simulink library "ammclib_bam_S32K3xx"  (R2016a)
(part 34 of 50)

      |   SampleTime=Simulink.data.evalinGlobal(bdroot,get_param(gcb,'SampleTime'));
      |   if (SampleTime==-1)
      |     SampleTime=str2double(get_param(gcb,'SampleTime_1'));
      |   end
      |   f16C1_bkup=get_param(gcb,'f16C1');
      |   u16NShift_bkup=get_param(gcb,'u16NShift');
      |   inscale=Simulink.data.evalinGlobal(bdroot,get_param(gcb,'inscale'));
      |   outscale=Simulink.data.evalinGlobal(bdroot,get_param(gcb,'outscale'));
      |   if (inscale<=0)
      |     warning('E_max must be positive.');
      |   end
      |   if (outscale<=0)
      |     warning('U_max must be positive.');
      |   end
      |   c1f=SampleTime*0.5*inscale/outscale;
      |   u16NShift=ceil(log2(abs(c1f)));
      |   if u16NShift<0
      |     u16NShift=0;
      |   end
      |   if u16NShift>15
      |     u16NShift=15;
      |     warning(['Parameter u16NShift of ' gcb ' exceeds the fixed-point range.']);
      |   end
      |   f16C1=round(c1f*2^(-u16NShift)*2^15);
      |   if f16C1>2^15-1
      |     f16C1=2^15-1;
      |     warning(['Parameter f16C1 of ' gcb ' exceeds the fixed-point range.']);
      |   end
      |   if f16C1<-2^15
      |     f16C1=-2^15;
      |     warning(['Parameter f16C1 of ' gcb ' exceeds the fixed-point range.']);
      |   end
      |   if isnan(f16C1)
      |     if ~strcmp(f16C1_bkup,'0')
      |       set_param(gcb,'f16C1','0');
      |     end
      |   else
      |     tmps=num2str(f16C1);
      |     if ~strcmp(f16C1_bkup,tmps)
      |       set_param(gcb,'f16C1',tmps);
      |     end
      |   end
      |   if isnan(u16NShift)
      |     if ~strcmp(u16NShift_bkup,'0')
      |       set_param(gcb,'u16NShift','0');
      |     end
      |   else
      |     tmps=num2str(u16NShift);
      |     if ~strcmp(u16NShift_bkup,tmps)
      |       set_param(gcb,'u16NShift',tmps);
      |     end
      |   end
      | end
      mask Callback autoCalcEn:
      | maskStr=get_param(gcb,'showStates');
      | if strcmp(maskStr,'Hide (faster execution)')
      |   p=Simulink.Mask.get(gcb);
      |   autoCalcEn=get_param(gcb,'autoCalcEn');
      |   hintText=p.getDialogControl('timeHint');
      |   if strcmp(autoCalcEn,'on')
      |     param=p.getParameter('outscale');
      |     if strcmp(param.Enabled,'off')
      |       SampleTime=Simulink.data.evalinGlobal(bdroot,get_param(gcb,'SampleTime'));
      |       if SampleTime==-1
      |         SampleTime=str2double(get_param(gcb,'SampleTime_1'));
      |         if isnan(SampleTime)
      |           hintText.Prompt=['Note: Implementation parameters cannot be calculated yet because the block''s inherited sample time is unknown. Simulink will update the sample time when you run the simulation.'];
      |         else
      |           hintText.Prompt=['Caution: Implementation parameters depend on inherited sample time. Make sure that the sample time of the block''s inputs corresponds to the sampling period in the target application.'];
      |         end
      |       else
      |         hintText.Prompt='Caution: Implementation parameters depend on the sample time. Make sure that the simulation time step corresponds to the sampling period in the target application.';
      |       end
      |       p=Simulink.Mask.get(gcb);
      |       param=p.getParameter('inscale');
      |       param.set('Enabled','on');
      |       param=p.getParameter('outscale');
      |       param.set('Enabled','on');
      |     else
      |       SampleTime=Simulink.data.evalinGlobal(bdroot,get_param(gcb,'SampleTime'));
      |       if SampleTime==-1
      |         SampleTime=str2double(get_param(gcb,'SampleTime_1'));
      |       end
      |     end
      |     f16C1_bkup=get_param(gcb,'f16C1');
      |     u16NShift_bkup=get_param(gcb,'u16NShift');
      |     inscale=Simulink.data.evalinGlobal(bdroot,get_param(gcb,'inscale'));
      |     outscale=Simulink.data.evalinGlobal(bdroot,get_param(gcb,'outscale'));
      |     if (inscale<=0)
      |       warning('E_max must be positive.');
      |     end
      |     if (outscale<=0)
      |       warning('U_max must be positive.');
      |     end
      |     c1f=SampleTime*0.5*inscale/outscale;
      |     u16NShift=ceil(log2(abs(c1f)));
      |     if u16NShift<0
      |       u16NShift=0;
      |     end
      |     if u16NShift>15
      |       u16NShift=15;
      |       warning(['Parameter u16NShift of ' gcb ' exceeds the fixed-point range.']);
      |     end
      |     f16C1=round(c1f*2^(-u16NShift)*2^15);
      |     if f16C1>2^15-1
      |       f16C1=2^15-1;
      |       warning(['Parameter f16C1 of ' gcb ' exceeds the fixed-point range.']);
      |     end
      |     if f16C1<-2^15
      |       f16C1=-2^15;
      |       warning(['Parameter f16C1 of ' gcb ' exceeds the fixed-point range.']);
      |     end
      |     if isnan(f16C1)
      |       if ~strcmp(f16C1_bkup,'0')
      |         set_param(gcb,'f16C1','0');
      |       end
      |     else
      |       tmps=num2str(f16C1);
      |       if ~strcmp(f16C1_bkup,tmps)
      |         set_param(gcb,'f16C1',tmps);
      |       end
      |     end
      |     if isnan(u16NShift)
      |       if ~strcmp(u16NShift_bkup,'0')
      |         set_param(gcb,'u16NShift','0');
      |       end
      |     else
      |       tmps=num2str(u16NShift);
      |       if ~strcmp(u16NShift_bkup,tmps)
      |         set_param(gcb,'u16NShift',tmps);
      |       end
      |     end
      |   else
      |     param=p.getParameter('outscale');
      |     if strcmp(param.Enabled,'on')
      |       hintText.Prompt='Caution: Implementation parameters are fixed.';
      |       p=Simulink.Mask.get(gcb);
      |       param=p.getParameter('inscale');
      |       param.set('Enabled','off');
      |       param=p.getParameter('outscale');
      |       param.set('Enabled','off');
      |     end
      |   end
      | end
      mask DialogControl CompBut Prompt: Recalculate sample times
      mask DialogControl CompBut Tooltip: Simulink updates the sample times of all blocks when the simulation is run. This button will update the sample times now.
      mask DialogControl CompBut Callback:
      | btn=questdlg('This will apply all changes in all open dialog boxes and update the schematic. Do you want to proceed?','Apply all changes','Continue','Cancel','Continue');
      | if strcmp(btn,'Continue')
      |   dlgs=DAStudio.ToolRoot.getOpenDialogs;
      |   for i=1:length(dlgs)
      |     dlgs(i).apply;
      |   end
      |   try
      |     SampleTime_1=str2double(get_param(gcb,'SampleTime_1'));
      |     ts=Simulink.Block.getSampleTimes(gcb);
      |     ts=ts(1).Value(1);
      |     if (SampleTime_1 ~= ts)
      |       SampleTime_1=ts;
      |       set_param(gcb,'SampleTime_1',num2str(ts));
      |       autoCalcEn=get_param(gcb,'autoCalcEn');
      |       if strcmp(autoCalcEn,'on')
      |         SampleTime=Simulink.data.evalinGlobal(bdroot,get_param(gcb,'SampleTime'));
      |         p=Simulink.Mask.get(gcb);
      |         hintText=p.getDialogControl('timeHint');
      |         if SampleTime==-1
      |           SampleTime=SampleTime_1;
      |           hintText.Prompt='Caution: Implementation parameters depend on inherited sample time. Make sure that the sample time of the block''s inputs corresponds to the sampling period in the target application.';
      |         else
      |           hintText.Prompt='Caution: Implementation parameters depend on the sample time. Make sure that the simulation time step corresponds to the sampling period in the target application.';
      |         end
      |         f16C1_bkup=get_param(gcb,'f16C1');
      |         u16NShift_bkup=get_param(gcb,'u16NShift');
      |         inscale=Simulink.data.evalinGlobal(bdroot,get_param(gcb,'inscale'));
      |         outscale=Simulink.data.evalinGlobal(bdroot,get_param(gcb,'outscale'));
      |         if (inscale<=0)
      |           warning('E_max must be positive.');
      |         end
      |         if (outscale<=0)
      |           warning('U_max must be positive.');
      |         end
      |         c1f=SampleTime*0.5*inscale/outscale;
      |         u16NShift=ceil(log2(abs(c1f)));
      |         if u16NShift<0
      |           u16NShift=0;
      |         end
      |         if u16NShift>15
      |           u16NShift=15;
      |           warning(['Parameter u16NShift of ' gcb ' exceeds the fixed-point range.']);
      |         end
      |         f16C1=round(c1f*2^(-u16NShift)*2^15);
      |         if f16C1>2^15-1
      |           f16C1=2^15-1;
      |           warning(['Parameter f16C1 of ' gcb ' exceeds the fixed-point range.']);
      |         end
      |         if f16C1<-2^15
      |           f16C1=-2^15;
      |           warning(['Parameter f16C1 of ' gcb ' exceeds the fixed-point range.']);
      |         end
      |         if isnan(f16C1)
      |           if ~strcmp(f16C1_bkup,'0')
      |             set_param(gcb,'f16C1','0');
      |           end
      |         else
      |           tmps=num2str(f16C1);
      |           if ~strcmp(f16C1_bkup,tmps)
      |             set_param(gcb,'f16C1',tmps);
      |           end
      |         end
      |         if isnan(u16NShift)
      |           if ~strcmp(u16NShift_bkup,'0')
      |             set_param(gcb,'u16NShift','0');
      |           end
      |         else
      |           tmps=num2str(u16NShift);
      |           if ~strcmp(u16NShift_bkup,tmps)
      |             set_param(gcb,'u16NShift',tmps);
      |           end
      |         end
      |       end
      |     end
      |   catch
      |    warning(['Sample time cannot be calculated for the block ' gcb])
      |   end
      | end
      mask DialogControl timeHint Prompt: Note: Implementation parameters cannot be calculated yet because the block's inherited sample time is unknown. Simulink will update the sample time when you run the simulation.
      mask Display:
      | color('black');
      | pos = get_param(gcb, 'Position');
      | width = pos(3) - pos(1);
      | height = pos(4) - pos(2);
      | tX=width/2;
      | tY=height - 25;
      | color('black');
      | text(tX,tY, 'GFLIB_IntegratorTR_F16', 'horizontalAlignment', 'center');
      | if showStates == 2
      |   color('red');
      |   text(tX,tY - 20, ['debugging mode' char(13) char(10) '(limited performance)'], 'horizontalAlignment', 'center');
      | end
  GFLIB_Limit_F16 : Subsystem  TreatAsAtomicUnit=on  mask(GFLIB_Limit_F16){showStates=Hide (faster execution), f16LowerLimit=0, f16UpperLimit=0}
      mask prompts: showStates "Show parameters as inputs:"; f16LowerLimit "f16LowerLimit (Lower limit):"; f16UpperLimit "f16UpperLimit (Upper limit):"
      mask help: Limit function in 16-bit fixed-point fractional implementation. Refer to the AMMCLIB User's Guide for further details.
      mask init:
      | ddName = get_param(bdroot,'DataDictionary');
      | if length(ddName)==0
      |   set_param(bdroot,'DataDictionary','ammclib_types.sldd');
      | else
      |   dd = Simulink.data.dictionary.open(ddName);
      |   data = getSection(dd,'Design Data');
      |   if ~exist(data,'SWLIBS_2Syst_F16')
      |     addDataSource(dd,'ammclib_types.sldd');
      |     saveChanges(dd);
      |   end
      | end
      | 
      | if showStates == 1
      |   % hidden state variables
      |   if strcmp(get_param([gcb '/f16LowerLimit'], 'BlockType'), 'Inport')
      |     posblk = get_param(gcb, 'Position');
      | 
      |     pos = get_param([gcb, '/f16LowerLimit'], 'Position');
      |     orient = get_param([gcb, '/f16LowerLimit'], 'Orientation');
      |     delete_block([gcb, '/f16LowerLimit']);
      |     add_block('built-in/Ground', [gcb, '/f16LowerLimit'], 'Position', pos, 'Orientation', orient);
      | 
      |     pos = get_param([gcb, '/f16UpperLimit'], 'Position');
      |     orient = get_param([gcb, '/f16UpperLimit'], 'Orientation');
      |     delete_block([gcb, '/f16UpperLimit']);
      |     add_block('built-in/Ground', [gcb, '/f16UpperLimit'], 'Position', pos, 'Orientation', orient);
      | 
      | 
      |     set_param([gcb '/f16In'], 'Port', '1');
      | 
      |     tmpOutCnt=0;
      |     tmpOutCnt=tmpOutCnt+1;
      |     set_param([gcb '/f16Out'], 'Port', num2str(tmpOutCnt));
      | 
      | set_param(gcb,'MaskEnables',{'on','on','on'});
      | 
      |     if (posblk(4) - posblk(2)) > 50
      |       height = 50;
      |       set_param(gcb,'Position',[posblk(1), posblk(2), posblk(3), posblk(2)+height])
      |     end
      |   end
      | else
      |   % shown state variables
      |   if strcmp(get_param([gcb '/f16LowerLimit'], 'BlockType'), 'Ground')
      |     posblk = get_param(gcb, 'Position');
      | 
      |     pos = get_param([gcb, '/f16LowerLimit'], 'Position');
      |     orient = get_param([gcb, '/f16LowerLimit'], 'Orientation');
      |     delete_block([gcb, '/f16LowerLimit']);
      |     add_block('built-in/Inport', [gcb, '/f16LowerLimit'], 'Position', pos, 'Orientation', orient, 'OutDataTypeStr', 'int16');
      | 
      |     pos = get_param([gcb, '/f16UpperLimit'], 'Position');
      |     orient = get_param([gcb, '/f16UpperLimit'], 'Orientation');
      |     delete_block([gcb, '/f16UpperLimit']);
      |     add_block('built-in/Inport', [gcb, '/f16UpperLimit'], 'Position', pos, 'Orientation', orient, 'OutDataTypeStr', 'int16');
      | 
      | 
      | 
      | 
      |     set_param([gcb '/f16In'], 'Port', '1');
      |     set_param([gcb '/f16LowerLimit'], 'Port', '2');
      |     set_param([gcb '/f16UpperLimit'], 'Port', '3');
      | 
      |     tmpOutCnt=0;
      |     tmpOutCnt=tmpOutCnt+1;
      |     set_param([gcb '/f16Out'], 'Port', num2str(tmpOutCnt));
      | 
      |     set_param(gcb,'MaskEnables',{'on','off','off'});
      | 
      |     if (posblk(4) - posblk(2)) < 100
      |       height = 100;
      |       set_param(gcb,'Position',[posblk(1), posblk(2), posblk(3), posblk(2)+height])
      |     end
      |   end
      | end
      settings: RTWSystemCode=Inline
      mask Help: web([fileparts(which('ammclib_bam_S32K3xx.slx')) '/../doc/S32K3XXMCLUG.pdf'], '-browser')
      mask TypeOptions showStates: Hide (faster execution) | Show (parameters can be changed during simulation)
      mask Callback showStates:
      | maskStr=get_param(gcb,'showStates');
      | if strcmp(maskStr,'Hide (faster execution)')
      |   if strcmp(get_param([gcb '/f16LowerLimit'], 'BlockType'), 'Inport')
      | set_param(gcb,'MaskEnables',{'on','on','on'});
      |   end
      | else
      |   if strcmp(get_param([gcb '/f16LowerLimit'], 'BlockType'), 'Ground')
      |     set_param(gcb,'MaskEnables',{'on','off','off'});
      |   end
      | end
      mask Display:
      | color('black');
      | pos = get_param(gcb, 'Position');
      | width = pos(3) - pos(1);
      | height = pos(4) - pos(2);
      | tX=width/2;
      | tY=height - 8;
      | color('black');
      | text(tX,tY, 'GFLIB_Limit_F16', 'horizontalAlignment', 'center');
      | if showStates == 2
      |   color('red');
      |   text(tX,tY - 20, ['debugging mode' char(13) char(10) '(limited performance)'], 'horizontalAlignment', 'center');
      | end
  GFLIB_LowerLimit_F16 : Subsystem  TreatAsAtomicUnit=on  mask(GFLIB_LowerLimit_F16){showStates=Hide (faster execution), f16LowerLimit=0}
      mask prompts: showStates "Show parameters as inputs:"; f16LowerLimit "f16LowerLimit (Value determining the lower limit threshold):"
      mask help: Lower limit function in 16-bit fixed-point fractional implementation. Refer to the AMMCLIB User's Guide for further details.
      mask init:
      | ddName = get_param(bdroot,'DataDictionary');
      | if length(ddName)==0
      |   set_param(bdroot,'DataDictionary','ammclib_types.sldd');
      | else
      |   dd = Simulink.data.dictionary.open(ddName);
      |   data = getSection(dd,'Design Data');
      |   if ~exist(data,'SWLIBS_2Syst_F16')
      |     addDataSource(dd,'ammclib_types.sldd');
      |     saveChanges(dd);
      |   end
      | end
      | 
      | if showStates == 1
      |   % hidden state variables
      |   if strcmp(get_param([gcb '/f16LowerLimit'], 'BlockType'), 'Inport')
      |     posblk = get_param(gcb, 'Position');
      | 
      |     pos = get_param([gcb, '/f16LowerLimit'], 'Position');
      |     orient = get_param([gcb, '/f16LowerLimit'], 'Orientation');
      |     delete_block([gcb, '/f16LowerLimit']);
      |     add_block('built-in/Ground', [gcb, '/f16LowerLimit'], 'Position', pos, 'Orientation', orient);
      | 
      | 
      |     set_param([gcb '/f16In'], 'Port', '1');
      | 
      |     tmpOutCnt=0;
      |     tmpOutCnt=tmpOutCnt+1;
      |     set_param([gcb '/f16Out'], 'Port', num2str(tmpOutCnt));
      | 
      | set_param(gcb,'MaskEnables',{'on','on'});
      | 
      |     if (posblk(4) - posblk(2)) > 50
      |       height = 50;
      |       set_param(gcb,'Position',[posblk(1), posblk(2), posblk(3), posblk(2)+height])
      |     end
      |   end
      | else
      |   % shown state variables
      |   if strcmp(get_param([gcb '/f16LowerLimit'], 'BlockType'), 'Ground')
      |     posblk = get_param(gcb, 'Position');
      | 
      |     pos = get_param([gcb, '/f16LowerLimit'], 'Position');
      |     orient = get_param([gcb, '/f16LowerLimit'], 'Orientation');
      |     delete_block([gcb, '/f16LowerLimit']);
      |     add_block('built-in/Inport', [gcb, '/f16LowerLimit'], 'Position', pos, 'Orientation', orient, 'OutDataTypeStr', 'int16');
      | 
      | 
      | 
      | 
      |     set_param([gcb '/f16In'], 'Port', '1');
      |     set_param([gcb '/f16LowerLimit'], 'Port', '2');
      | 
      |     tmpOutCnt=0;
      |     tmpOutCnt=tmpOutCnt+1;
      |     set_param([gcb '/f16Out'], 'Port', num2str(tmpOutCnt));
      | 
      |     set_param(gcb,'MaskEnables',{'on','off'});
      | 
      |     if (posblk(4) - posblk(2)) < 75
      |       height = 75;
      |       set_param(gcb,'Position',[posblk(1), posblk(2), posblk(3), posblk(2)+height])
      |     end
      |   end
      | end
      settings: RTWSystemCode=Inline
      mask Help: web([fileparts(which('ammclib_bam_S32K3xx.slx')) '/../doc/S32K3XXMCLUG.pdf'], '-browser')
      mask TypeOptions showStates: Hide (faster execution) | Show (parameters can be changed during simulation)
      mask Callback showStates:
      | maskStr=get_param(gcb,'showStates');
      | if strcmp(maskStr,'Hide (faster execution)')
      |   if strcmp(get_param([gcb '/f16LowerLimit'], 'BlockType'), 'Inport')
      | set_param(gcb,'MaskEnables',{'on','on'});
      |   end
      | else
      |   if strcmp(get_param([gcb '/f16LowerLimit'], 'BlockType'), 'Ground')
      |     set_param(gcb,'MaskEnables',{'on','off'});
      |   end
      | end
      mask Display:
      | color('black');
      | pos = get_param(gcb, 'Position');
      | width = pos(3) - pos(1);
      | height = pos(4) - pos(2);
      | tX=width/2;
      | tY=height - 8;
      | color('black');
      | text(tX,tY, 'GFLIB_LowerLimit_F16', 'horizontalAlignment', 'center');
      | if showStates == 2
      |   color('red');
      |   text(tX,tY - 20, ['debugging mode' char(13) char(10) '(limited performance)'], 'horizontalAlignment', 'center');
      | end
  GFLIB_Lut1D_F16 : Subsystem  TreatAsAtomicUnit=on  mask(GFLIB_Lut1D_F16){pf16Table=2^15*[-0.75 -0.25 0.0 0.25 0.75], s16MidIdx=2}
      mask prompts: pf16Table "pf16Table (Vector holding the ordinate values of interpolating intervals):"; s16MidIdx "Middle index in the table (zero-based indexing). This index is added to pf16Table to allow shifting the origin of the table to any point within the table:"
      mask help: One dimensional lookup table function in 16-bit fixed-point fractional implementation. Refer to the AMMCLIB User's Guide for further details.
      mask init: same as ammclib_bam_S32K3xx/GDFLIB/F16/GDFLIB_FilterFIR_F16
      settings: RTWSystemCode=Inline
      mask Help: web([fileparts(which('ammclib_bam_S32K3xx.slx')) '/../doc/S32K3XXMCLUG.pdf'], '-browser')
      mask Display: pos = get_param(gcb, 'Position');width = pos(3) - pos(1); height = pos(4) - pos(2);tX=width/2;tY=height - 8;color('black');text(tX,tY, 'GFLIB_Lut1D_F16', 'horizontalAlignment', 'center');
  GFLIB_Lut2D_F16 : Subsystem  TreatAsAtomicUnit=on  mask(GFLIB_Lut2D_F16){pf16Table=2^15*[-0.75 0.0 0.75; -0.5 0.0 0.5; -0.25 0.0 0.25], s16MidIdx=4}
      mask prompts: pf16Table "pf16Table (Matrix of z-coordinate values at vertices):"; s16MidIdx "Middle index in the table (zero-based indexing over all elements). This index is added to pf16Table to allow shifting the origin of the table coordinates to any point within the table:"
      mask help: Two dimensional lookup table function in 16-bit fixed-point fractional implementation. Refer to the AMMCLIB User's Guide for further details.
      mask init: same as ammclib_bam_S32K3xx/GDFLIB/F16/GDFLIB_FilterFIR_F16
      settings: RTWSystemCode=Inline
      mask Help: web([fileparts(which('ammclib_bam_S32K3xx.slx')) '/../doc/S32K3XXMCLUG.pdf'], '-browser')
      mask Display: pos = get_param(gcb, 'Position');width = pos(3) - pos(1); height = pos(4) - pos(2);tX=width/2;tY=height - 8;color('black');text(tX,tY, 'GFLIB_Lut2D_F16', 'horizontalAlignment', 'center');
  GFLIB_Ramp_F16 : Subsystem  TreatAsAtomicUnit=on  mask(GFLIB_Ramp_F16){showStates=Hide (faster execution), f16RampUp=0, f16RampDown=0}
      mask prompts: showStates "Show internal states:"; f16RampUp "f16RampUp (Ramp up increment coefficient):"; f16RampDown "f16RampDown (Ramp decrement coefficient):"
      mask help: Rate of change limiter - ramp function in 16-bit fixed-point fractional implementation. Refer to the AMMCLIB User's Guide for further details.
      mask init:
      | ddName = get_param(bdroot,'DataDictionary');
      | if length(ddName)==0
      |   set_param(bdroot,'DataDictionary','ammclib_types.sldd');
      | else
      |   dd = Simulink.data.dictionary.open(ddName);
      |   data = getSection(dd,'Design Data');
      |   if ~exist(data,'SWLIBS_2Syst_F16')
      |     addDataSource(dd,'ammclib_types.sldd');
      |     saveChanges(dd);
      |   end
      | end
      | 
      | if showStates == 1
      |   % hidden state variables
      |   if strcmp(get_param([gcb '/f16State'], 'BlockType'), 'Inport')
      |     posblk = get_param(gcb, 'Position');
      | 
      |     pos = get_param([gcb, '/f16State'], 'Position');
      |     orient = get_param([gcb, '/f16State'], 'Orientation');
      |     delete_block([gcb, '/f16State']);
      |     add_block('built-in/Ground', [gcb, '/f16State'], 'Position', pos, 'Orientation', orient);
      | 
      |     pos = get_param([gcb, '/f16RampUp'], 'Position');
      |     orient = get_param([gcb, '/f16RampUp'], 'Orientation');
      |     delete_block([gcb, '/f16RampUp']);
      |     add_block('built-in/Ground', [gcb, '/f16RampUp'], 'Position', pos, 'Orientation', orient);
      | 
      |     pos = get_param([gcb, '/f16RampDown'], 'Position');
      |     orient = get_param([gcb, '/f16RampDown'], 'Orientation');
      |     delete_block([gcb, '/f16RampDown']);
      |     add_block('built-in/Ground', [gcb, '/f16RampDown'], 'Position', pos, 'Orientation', orient);
      | 
      | 
      |     pos = get_param([gcb '/f16State_Out'], 'Position');
      |     orient = get_param([gcb '/f16State_Out'], 'Orientation');
      |     delete_block([gcb '/f16State_Out']);
      |     add_block('built-in/Terminator', [gcb '/f16State_Out'], 'Position', pos, 'Orientation', orient);
      | 
      |     set_param([gcb '/f16In'], 'Port', '1');
      | 
      |     tmpOutCnt=0;
      |     tmpOutCnt=tmpOutCnt+1;
      |     set_param([gcb '/f16Out'], 'Port', num2str(tmpOutCnt));
      | 
      | set_param(gcb,'MaskEnables',{'on','on','on'});
      | 
      |     if (posblk(4) - posblk(2)) > 50
      |       height = 50;
      |       set_param(gcb,'Position',[posblk(1), posblk(2), posblk(3), posblk(2)+height])
      |     end
      |   end
      | else
      |   % shown state variables
      |   if strcmp(get_param([gcb '/f16State'], 'BlockType'), 'Ground')
      |     posblk = get_param(gcb, 'Position');
      | 
      |     pos = get_param([gcb, '/f16State'], 'Position');
      |     orient = get_param([gcb, '/f16State'], 'Orientation');
      |     delete_block([gcb, '/f16State']);
      |     add_block('built-in/Inport', [gcb, '/f16State'], 'Position', pos, 'Orientation', orient, 'OutDataTypeStr', 'int16');
      | 
      |     pos = get_param([gcb, '/f16RampUp'], 'Position');
      |     orient = get_param([gcb, '/f16RampUp'], 'Orientation');
      |     delete_block([gcb, '/f16RampUp']);
      |     add_block('built-in/Inport', [gcb, '/f16RampUp'], 'Position', pos, 'Orientation', orient, 'OutDataTypeStr', 'int16');
      | 
      |     pos = get_param([gcb, '/f16RampDown'], 'Position');
      |     orient = get_param([gcb, '/f16RampDown'], 'Orientation');
      |     delete_block([gcb, '/f16RampDown']);
      |     add_block('built-in/Inport', [gcb, '/f16RampDown'], 'Position', pos, 'Orientation', orient, 'OutDataTypeStr', 'int16');
      | 
      | 
      | 
      |     pos = get_param([gcb '/f16State_Out'], 'Position');
      |     orient = get_param([gcb '/f16State_Out'], 'Orientation');
      |     delete_block([gcb '/f16State_Out']);
      |     add_block('built-in/Outport', [gcb '/f16State_Out'], 'Position', pos, 'Orientation', orient);
      | 
      | 
      |     set_param([gcb '/f16In'], 'Port', '1');
      |     set_param([gcb '/f16State'], 'Port', '2');
      |     set_param([gcb '/f16RampUp'], 'Port', '3');
      |     set_param([gcb '/f16RampDown'], 'Port', '4');
      | 
      |     tmpOutCnt=0;
      |     tmpOutCnt=tmpOutCnt+1;
      |     set_param([gcb '/f16Out'], 'Port', num2str(tmpOutCnt));
      |     tmpOutCnt=tmpOutCnt+1;
      |     set_param([gcb '/f16State_Out'], 'Port', num2str(tmpOutCnt));
      | 
      |     set_param(gcb,'MaskEnables',{'on','off','off'});
      | 
      |     if (posblk(4) - posblk(2)) < 125
      |       height = 125;
      |       set_param(gcb,'Position',[posblk(1), posblk(2), posblk(3), posblk(2)+height])
      |     end
      |   end
      | end
      settings: RTWSystemCode=Inline
      mask Help: web([fileparts(which('ammclib_bam_S32K3xx.slx')) '/../doc/S32K3XXMCLUG.pdf'], '-browser')
      mask TypeOptions showStates: Hide (faster execution) | Show (allows debugging; connect feedback loops manually)
      mask Callback showStates:
      | maskStr=get_param(gcb,'showStates');
      | if strcmp(maskStr,'Hide (faster execution)')
      |   if strcmp(get_param([gcb '/f16State'], 'BlockType'), 'Inport')
      | set_param(gcb,'MaskEnables',{'on','on','on'});
      |   end
      | else
      |   if strcmp(get_param([gcb '/f16State'], 'BlockType'), 'Ground')
      |     set_param(gcb,'MaskEnables',{'on','off','off'});
      |   end
      | end
      mask Display:
      | color('black');
      | pos = get_param(gcb, 'Position');
      | width = pos(3) - pos(1);
      | height = pos(4) - pos(2);
      | tX=width/2;
      | tY=height - 8;
      | color('black');
      | text(tX,tY, 'GFLIB_Ramp_F16', 'horizontalAlignment', 'center');
      | if showStates == 2
      |   color('red');
      |   text(tX,tY - 20, ['debugging mode' char(13) char(10) '(limited performance)'], 'horizontalAlignment', 'center');
      | end
  GFLIB_Sign_F16 : Subsystem  TreatAsAtomicUnit=on  mask(GFLIB_Sign_F16){}
      mask help: Bit accurate model of GFLIB_Sign function in 16-bit fixed-point fractional implementation. Refer to the AMMCLIB User's Guide for further details.
      mask init: same as ammclib_bam_S32K3xx/GDFLIB/F16/GDFLIB_FilterFIR_F16
      settings: RTWSystemCode=Inline
      mask Help: web([fileparts(which('ammclib_bam_S32K3xx.slx')) '/../doc/S32K3XXMCLUG.pdf'], '-browser')
      mask Display: pos = get_param(gcb, 'Position');width = pos(3) - pos(1); height = pos(4) - pos(2);tX=width/2;tY=height - 8;color('black');text(tX,tY, 'GFLIB_Sign_F16', 'horizontalAlignment', 'center');
  GFLIB_SinCos_F16 : Subsystem  TreatAsAtomicUnit=on  mask(GFLIB_SinCos_F16){}
      mask help: Calculation of sine and cosine of the same argument in 16-bit fixed-point fractional implementation. Refer to the AMMCLIB User's Guide for further details.
      mask init: same as ammclib_bam_S32K3xx/GDFLIB/F16/GDFLIB_FilterFIR_F16
      settings: RTWSystemCode=Inline
      mask Help: web([fileparts(which('ammclib_bam_S32K3xx.slx')) '/../doc/S32K3XXMCLUG.pdf'], '-browser')
      mask Display: pos = get_param(gcb, 'Position');width = pos(3) - pos(1); height = pos(4) - pos(2);tX=width/2;tY=height - 8;color('black');text(tX,tY, 'GFLIB_SinCos_F16', 'horizontalAlignment', 'center');
  GFLIB_Sin_F16 : Subsystem  TreatAsAtomicUnit=on  mask(GFLIB_Sin_F16){}
      mask help: Sine function in 16-bit fixed-point fractional implementation. Refer to the AMMCLIB User's Guide for further details.
      mask init: same as ammclib_bam_S32K3xx/GDFLIB/F16/GDFLIB_FilterFIR_F16
      settings: RTWSystemCode=Inline
      mask Help: web([fileparts(which('ammclib_bam_S32K3xx.slx')) '/../doc/S32K3XXMCLUG.pdf'], '-browser')
      mask Display: pos = get_param(gcb, 'Position');width = pos(3) - pos(1); height = pos(4) - pos(2);tX=width/2;tY=height - 8;color('black');text(tX,tY, 'GFLIB_Sin_F16', 'horizontalAlignment', 'center');
  GFLIB_Sqrt_F16 : Subsystem  TreatAsAtomicUnit=on  mask(GFLIB_Sqrt_F16){}
      mask help: Square root approximation in 16-bit fixed-point fractional implementation. Refer to the AMMCLIB User's Guide for further details.
      mask init: same as ammclib_bam_S32K3xx/GDFLIB/F16/GDFLIB_FilterFIR_F16
      settings: RTWSystemCode=Inline
      mask Help: web([fileparts(which('ammclib_bam_S32K3xx.slx')) '/../doc/S32K3XXMCLUG.pdf'], '-browser')
      mask Display: pos = get_param(gcb, 'Position');width = pos(3) - pos(1); height = pos(4) - pos(2);tX=width/2;tY=height - 8;color('black');text(tX,tY, 'GFLIB_Sqrt_F16', 'horizontalAlignment', 'center');
  GFLIB_Tan_F16 : Subsystem  TreatAsAtomicUnit=on  mask(GFLIB_Tan_F16){}
      mask help: Tangent function in 16-bit fixed-point fractional implementation. Refer to the AMMCLIB User's Guide for further details.
      mask init: same as ammclib_bam_S32K3xx/GDFLIB/F16/GDFLIB_FilterFIR_F16
      settings: RTWSystemCode=Inline
      mask Help: web([fileparts(which('ammclib_bam_S32K3xx.slx')) '/../doc/S32K3XXMCLUG.pdf'], '-browser')
      mask Display: pos = get_param(gcb, 'Position');width = pos(3) - pos(1); height = pos(4) - pos(2);tX=width/2;tY=height - 8;color('black');text(tX,tY, 'GFLIB_Tan_F16', 'horizontalAlignment', 'center');
  GFLIB_UpperLimit_F16 : Subsystem  TreatAsAtomicUnit=on  mask(GFLIB_UpperLimit_F16){showStates=Hide (faster execution), f16UpperLimit=0}
      mask prompts: showStates "Show parameters as inputs:"; f16UpperLimit "f16UpperLimit (Value determining the upper limit threshold):"
      mask help: Upper limit function in 16-bit fixed-point fractional implementation. Refer to the AMMCLIB User's Guide for further details.
      mask init:
      | ddName = get_param(bdroot,'DataDictionary');
      | if length(ddName)==0
      |   set_param(bdroot,'DataDictionary','ammclib_types.sldd');
      | else
      |   dd = Simulink.data.dictionary.open(ddName);
      |   data = getSection(dd,'Design Data');
      |   if ~exist(data,'SWLIBS_2Syst_F16')
      |     addDataSource(dd,'ammclib_types.sldd');
      |     saveChanges(dd);
      |   end
      | end
      | 
      | if showStates == 1
      |   % hidden state variables
      |   if strcmp(get_param([gcb '/f16UpperLimit'], 'BlockType'), 'Inport')
      |     posblk = get_param(gcb, 'Position');
      | 
      |     pos = get_param([gcb, '/f16UpperLimit'], 'Position');
      |     orient = get_param([gcb, '/f16UpperLimit'], 'Orientation');
      |     delete_block([gcb, '/f16UpperLimit']);
      |     add_block('built-in/Ground', [gcb, '/f16UpperLimit'], 'Position', pos, 'Orientation', orient);
      | 
      | 
      |     set_param([gcb '/f16In'], 'Port', '1');
      | 
      |     tmpOutCnt=0;
      |     tmpOutCnt=tmpOutCnt+1;
      |     set_param([gcb '/f16Out'], 'Port', num2str(tmpOutCnt));
      | 
      | set_param(gcb,'MaskEnables',{'on','on'});
      | 
      |     if (posblk(4) - posblk(2)) > 50
      |       height = 50;
      |       set_param(gcb,'Position',[posblk(1), posblk(2), posblk(3), posblk(2)+height])
      |     end
      |   end
      | else
      |   % shown state variables
      |   if strcmp(get_param([gcb '/f16UpperLimit'], 'BlockType'), 'Ground')
      |     posblk = get_param(gcb, 'Position');
      | 
      |     pos = get_param([gcb, '/f16UpperLimit'], 'Position');
      |     orient = get_param([gcb, '/f16UpperLimit'], 'Orientation');
      |     delete_block([gcb, '/f16UpperLimit']);
      |     add_block('built-in/Inport', [gcb, '/f16UpperLimit'], 'Position', pos, 'Orientation', orient, 'OutDataTypeStr', 'int16');
      | 
      | 
      | 
      | 
      |     set_param([gcb '/f16In'], 'Port', '1');
      |     set_param([gcb '/f16UpperLimit'], 'Port', '2');
      | 
      |     tmpOutCnt=0;
      |     tmpOutCnt=tmpOutCnt+1;
      |     set_param([gcb '/f16Out'], 'Port', num2str(tmpOutCnt));
      | 
      |     set_param(gcb,'MaskEnables',{'on','off'});
      | 
      |     if (posblk(4) - posblk(2)) < 75
      |       height = 75;
      |       set_param(gcb,'Position',[posblk(1), posblk(2), posblk(3), posblk(2)+height])
      |     end
      |   end
      | end
      settings: RTWSystemCode=Inline
      mask Help: web([fileparts(which('ammclib_bam_S32K3xx.slx')) '/../doc/S32K3XXMCLUG.pdf'], '-browser')
      mask TypeOptions showStates: Hide (faster execution) | Show (parameters can be changed during simulation)
      mask Callback showStates:
      | maskStr=get_param(gcb,'showStates');
      | if strcmp(maskStr,'Hide (faster execution)')
      |   if strcmp(get_param([gcb '/f16UpperLimit'], 'BlockType'), 'Inport')
      | set_param(gcb,'MaskEnables',{'on','on'});
      |   end
      | else
      |   if strcmp(get_param([gcb '/f16UpperLimit'], 'BlockType'), 'Ground')
      |     set_param(gcb,'MaskEnables',{'on','off'});
      |   end
      | end
      mask Display:
      | color('black');
      | pos = get_param(gcb, 'Position');
      | width = pos(3) - pos(1);
      | height = pos(4) - pos(2);
      | tX=width/2;
      | tY=height - 8;
      | color('black');
      | text(tX,tY, 'GFLIB_UpperLimit_F16', 'horizontalAlignment', 'center');
      | if showStates == 2
      |   color('red');
      |   text(tX,tY - 20, ['debugging mode' char(13) char(10) '(limited performance)'], 'horizontalAlignment', 'center');
      | end
  GFLIB_VMin_F16 : Subsystem  TreatAsAtomicUnit=on  mask(GFLIB_VMin_F16){}
      mask help: 16-bit fixed-point implementation of the GFLIB_VMin function, which finds the index of a vector minimum. Refer to the AMMCLIB User's Guide for further details.
      mask init: same as ammclib_bam_S32K3xx/GDFLIB/F16/GDFLIB_FilterFIR_F16
      settings: RTWSystemCode=Inline
      mask Help: web([fileparts(which('ammclib_bam_S32K3xx.slx')) '/../doc/S32K3XXMCLUG.pdf'], '-browser')
      mask Display: pos = get_param(gcb, 'Position');width = pos(3) - pos(1); height = pos(4) - pos(2);tX=width/2;tY=height - 8;color('black');text(tX,tY, 'GFLIB_VMin_F16', 'horizontalAlignment', 'center');
  GFLIB_VectorLimit_F16 : Subsystem  TreatAsAtomicUnit=on  mask(GFLIB_VectorLimit_F16){showStates=Hide (faster execution), f16Limit=0}
      mask prompts: showStates "Show parameters as inputs:"; f16Limit "f16Limit (The maximum magnitude of the input 2-element vector):"
      mask help: 16-bit fixed-point fractional implementation of the GFLIB_VectorLimit function which limits the magnitude of the input 2-element vector, keeping its direction unchanged. Refer to the AMMCLIB User's Guide for further details.
      mask init:
      | ddName = get_param(bdroot,'DataDictionary');
      | if length(ddName)==0
      |   set_param(bdroot,'DataDictionary','ammclib_types.sldd');
      | else
      |   dd = Simulink.data.dictionary.open(ddName);
      |   data = getSection(dd,'Design Data');
      |   if ~exist(data,'SWLIBS_2Syst_F16')
      |     addDataSource(dd,'ammclib_types.sldd');
      |     saveChanges(dd);
      |   end
      | end
      | 
      | if showStates == 1
      |   % hidden state variables
      |   if strcmp(get_param([gcb '/f16Limit'], 'BlockType'), 'Inport')
      |     posblk = get_param(gcb, 'Position');
      | 
      |     pos = get_param([gcb, '/f16Limit'], 'Position');
      |     orient = get_param([gcb, '/f16Limit'], 'Orientation');
      |     delete_block([gcb, '/f16Limit']);
      |     add_block('built-in/Ground', [gcb, '/f16Limit'], 'Position', pos, 'Orientation', orient);
      | 
      | 
      |     set_param([gcb '/pIn'], 'Port', '1');
      | 
      |     tmpOutCnt=0;
      |     tmpOutCnt=tmpOutCnt+1;
      |     set_param([gcb '/bFlag'], 'Port', num2str(tmpOutCnt));
      |     tmpOutCnt=tmpOutCnt+1;
      |     set_param([gcb '/pOut'], 'Port', num2str(tmpOutCnt));
      | 
      | set_param(gcb,'MaskEnables',{'on','on'});
      | 
      |     if (posblk(4) - posblk(2)) > 75
      |       height = 75;
      |       set_param(gcb,'Position',[posblk(1), posblk(2), posblk(3), posblk(2)+height])
      |     end
      |   end
      | else
      |   % shown state variables
      |   if strcmp(get_param([gcb '/f16Limit'], 'BlockType'), 'Ground')
      |     posblk = get_param(gcb, 'Position');
      | 
      |     pos = get_param([gcb, '/f16Limit'], 'Position');
      |     orient = get_param([gcb, '/f16Limit'], 'Orientation');
      |     delete_block([gcb, '/f16Limit']);
      |     add_block('built-in/Inport', [gcb, '/f16Limit'], 'Position', pos, 'Orientation', orient, 'OutDataTypeStr', 'int16');
      | 
      | 
      | 
      | 
      |     set_param([gcb '/pIn'], 'Port', '1');
      |     set_param([gcb '/f16Limit'], 'Port', '2');
      | 
      |     tmpOutCnt=0;
      |     tmpOutCnt=tmpOutCnt+1;
      |     set_param([gcb '/bFlag'], 'Port', num2str(tmpOutCnt));
      |     tmpOutCnt=tmpOutCnt+1;
      |     set_param([gcb '/pOut'], 'Port', num2str(tmpOutCnt));
      | 
      |     set_param(gcb,'MaskEnables',{'on','off'});
      | 
      |     if (posblk(4) - posblk(2)) < 75
      |       height = 75;
      |       set_param(gcb,'Position',[posblk(1), posblk(2), posblk(3), posblk(2)+height])
      |     end
      |   end
      | end
      settings: RTWSystemCode=Inline
      mask Help: web([fileparts(which('ammclib_bam_S32K3xx.slx')) '/../doc/S32K3XXMCLUG.pdf'], '-browser')
      mask TypeOptions showStates: Hide (faster execution) | Show (parameters can be changed during simulation)
      mask Callback showStates:
      | maskStr=get_param(gcb,'showStates');
      | if strcmp(maskStr,'Hide (faster execution)')
      |   if strcmp(get_param([gcb '/f16Limit'], 'BlockType'), 'Inport')
      | set_param(gcb,'MaskEnables',{'on','on'});
      |   end
      | else
      |   if strcmp(get_param([gcb '/f16Limit'], 'BlockType'), 'Ground')
      |     set_param(gcb,'MaskEnables',{'on','off'});
      |   end
      | end
      mask Display:
      | color('black');
      | pos = get_param(gcb, 'Position');
      | width = pos(3) - pos(1);
      | height = pos(4) - pos(2);
      | tX=width/2;
      | tY=height - 8;
      | color('black');
      | text(tX,tY, 'GFLIB_VectorLimit_F16', 'horizontalAlignment', 'center');
      | if showStates == 2
      |   color('red');
      |   text(tX,tY - 20, ['debugging mode' char(13) char(10) '(limited performance)'], 'horizontalAlignment', 'center');
      | end
